simulink model "Mdl_Examle03"  (Simulink 6.1)
settings: Solver=ode4  StartTime=0.0  StopTime=2  FixedStep=0.01  RelTol=1e-3
values from neighbouring files (symbols this model uses):
  A = [1 0 0;3 -1 1;0 2 0]    [Example03.m]
  B = [2 1 1]'    [Example03.m]
  C = [0 0 1]    [Example03.m]
  F = A11_bar-L*A21_bar    [Example03.m]
  G = (A11_bar-L*A21_bar)*L+A12_bar-L*A22_bar    [Example03.m]
  H = B1_bar-L*B2_bar    [Example03.m]
  Q = [1 0 0;0 1 0;0 0 1]    [Example03.m]
undefined symbols (not defined in the file or in its folder): AA, BB
settings Model: LastModifiedBy=ybstrong
settings DebuggingCC: SolverPrmCheckMsg=warning

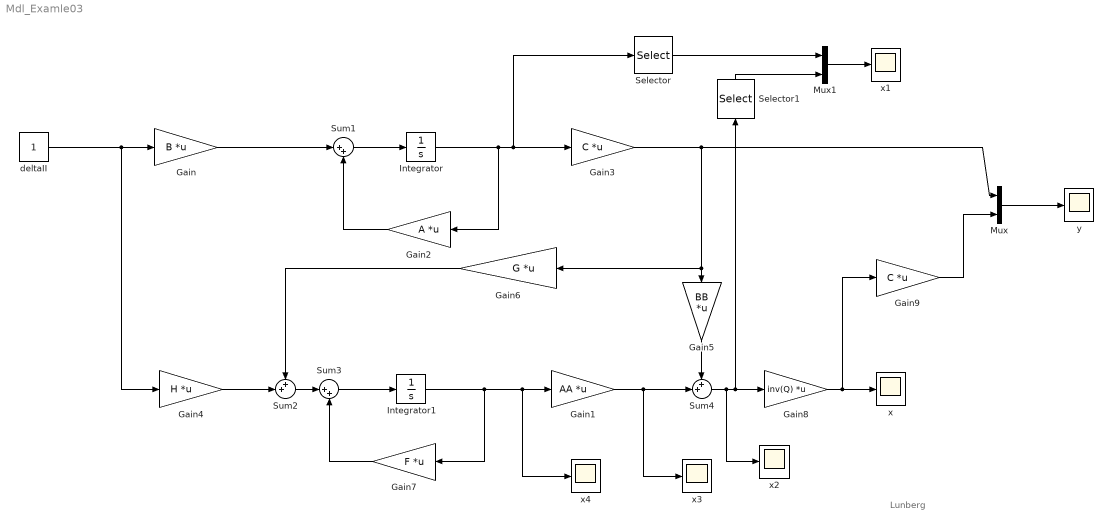
== system Mdl_Examle03 ==
  note: Lunberg
  Gain : Gain  Gain=B  Multiplication=Matrix(K*u)
  Gain1 : Gain  Gain=AA  Multiplication=Matrix(K*u)
  Gain2 : Gain  Orientation=left  Gain=A  Multiplication=Matrix(K*u)
  Gain3 : Gain  Gain=C  Multiplication=Matrix(K*u)
  Gain4 : Gain  Gain=H  Multiplication=Matrix(K*u)
  Gain5 : Gain  Orientation=down  Gain=BB  Multiplication=Matrix(K*u)
  Gain6 : Gain  Orientation=left  Gain=G  Multiplication=Matrix(K*u)
  Gain7 : Gain  Orientation=left  Gain=F  Multiplication=Matrix(K*u)
  Gain8 : Gain  Gain=inv(Q)  Multiplication=Matrix(K*u)
  Gain9 : Gain  Gain=C  Multiplication=Matrix(K*u)
  Integrator : Integrator  InitialCondition=[0;1;2]
  Integrator1 : Integrator
  Mux : Mux  Inputs=2
  Mux1 : Mux  Inputs=2
  Selector : Selector  Elements=3  InputPortWidth=3
  Selector1 : Selector  Orientation=up  Elements=3  InputPortWidth=3
  Sum1 : Sum  Inputs=|++
  Sum2 : Sum  Inputs=++|
  Sum3 : Sum  Inputs=|++
  Sum4 : Sum  Inputs=++|
  deltaII : Constant
  x{,1..4} (5 alike) : Scope
      x1 settings: SaveName=ScopeData2
      x2 settings: SaveName=ScopeData3
      x3 settings: SaveName=ScopeData4
      x4 settings: SaveName=ScopeData5
  y : Scope
  wires:
  deltaII/1 -> Gain/1, Gain4/1
  Gain/1 -> Sum1/1
  Sum1/1 -> Integrator/1
  Integrator/1 -> Gain2/1, Gain3/1, Selector/1
  Gain2/1 -> Sum1/2
  Gain3/1 -> Gain6/1, Gain5/1, Mux/1
  Gain4/1 -> Sum2/2
  Sum2/1 -> Sum3/1
  Integrator1/1 -> Gain7/1, Gain1/1, x4/1
  Sum3/1 -> Integrator1/1
  Gain1/1 -> Sum4/2, x3/1
  Gain7/1 -> Sum3/2
  Gain6/1 -> Sum2/1
  Gain5/1 -> Sum4/1
  Sum4/1 -> Gain8/1, Selector1/1, x2/1
  Gain8/1 -> x/1, Gain9/1
  Gain9/1 -> Mux/2
  Mux/1 -> y/1
  Mux1/1 -> x1/1
  Selector/1 -> Mux1/1
  Selector1/1 -> Mux1/2
